simulink model "wiper_mechanism_for_from_workspace"  (R2020a)
settings: Solver=FixedStepDiscrete  StartTime=0.0  StopTime=50  FixedStep=1  RelTol=1e-3
settings Model: Creator=Kundan Patil  LastModifiedBy=Kundan Patil
settings OptimizationCC: DefaultParameterBehavior=Inlined  EnhancedBackFolding=on  PassReuseOutputArgsAs=Individual arguments  ZeroExternalMemoryAtStartup=off  ZeroInternalMemoryAtStartup=off  OptimizeBlockOrder=speed  DifferentSizesBufferReuse=on  OptimizationCustomize=off  EfficientTunableParamExpr=on
settings DebuggingCC: ParameterTunabilityLossMsg=error
settings SFSimCC: MATLABDynamicMemAlloc=off
settings RTWCC: SystemTargetFile=ert.tlc  GenCodeOnly=on  TemplateMakefile=ert_default_tmf  GenerateReport=on  IncludeHyperlinkInReport=on  LaunchReport=on  GenerateTraceInfo=on  GenerateWebview=on
settings CodeAppCC: ForceParamTrailComments=on  IgnoreCustomStorageClasses=off  OperatorAnnotations=on  SimulinkDataObjDesc=on  SFDataObjDesc=on  InsertBlockDesc=on
settings ERTTargetCC: TargetLangStandard=C99 (ISO)  GenerateSampleERTMain=on  InlinedParameterPlacement=NonHierarchical  ERTCustomFileTemplate=example_file_process.tlc

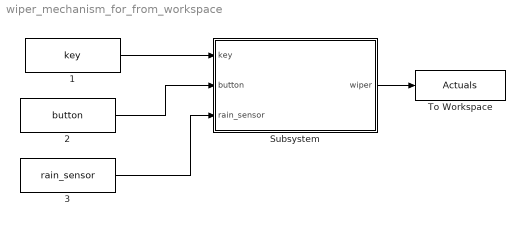
== system wiper_mechanism_for_from_workspace ==
  1 : FromWorkspace  VariableName=key
  2 : FromWorkspace  VariableName=button
  3 : FromWorkspace  VariableName=rain_sensor
  Subsystem : Subsystem
  To Workspace : ToWorkspace  VariableName=Actuals  SaveFormat=Timeseries  SampleTime=-1
  wires:
  1/1 -> Subsystem/1(key)
  2/1 -> Subsystem/2(button)
  3/1 -> Subsystem/3(rain_sensor)
  Subsystem/1(wiper) -> To Workspace/1

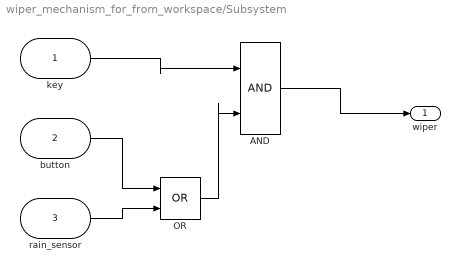
== system wiper_mechanism_for_from_workspace/Subsystem ==
  key : Inport
  button : Inport  Port=2
  rain_sensor : Inport  Port=3
  AND : Logic  IconShape=distinctive  AllPortsSameDT=off  OutDataTypeStr=boolean
  OR : Logic  Operator=OR  IconShape=distinctive  AllPortsSameDT=off  OutDataTypeStr=boolean
  wiper : Outport
  wires:
  key/1 -> AND/1
  AND/1 -> wiper/1
  rain_sensor/1 -> OR/2
  OR/1 -> AND/2
  button/1 -> OR/1
